simulink model "UNIFIER_ROMdyn_slx"  (R2023b)
settings: Solver=VariableStepAuto  StartTime=0.0  StopTime=0  RelTol=1e-3
InitFcn:
  | UNIFIER_LOAD_ROM
values from neighbouring files (symbols this model uses):
  c = 1.43676    [UNIFIER_LOAD.mat]
  dp_DEP =     [UNIFIER_LOAD.mat]
  dp_HTU =     [UNIFIER_LOAD.mat]
  m = 7057    [UNIFIER_LOAD.mat]
  S = 29.98388    [UNIFIER_LOAD.mat]
  xyz_DEP = [-6.9629998 -10.05 -0.90899998 -6.921 -8.4499998 -0.792 -6.8660002 -6.8499999 -0.82300001 -6.8099999 -5.25 -0.85000002 ... (36 elements, 3x12)]    [UNIFIER_LOAD.mat]
undefined symbols (not defined in the file or in its folder): g, Iyy, ROM, xyz_cg_12
libraries: dspindex x2, simulink x1, aerolibatmos2 x1
settings Model: Creator=Reggie Johanes  LastModifiedBy=Reggie Johanes

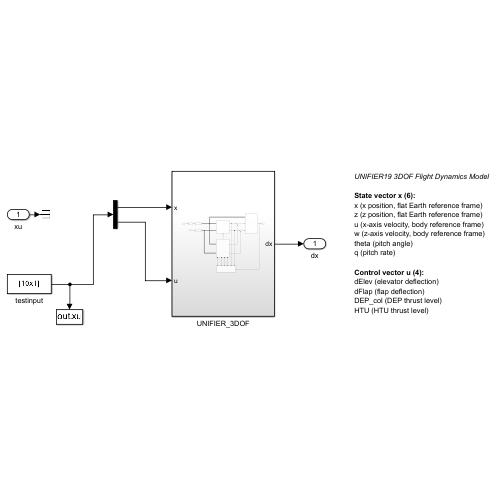
[thumbnail: Simulink's stored preview of the top-level diagram]
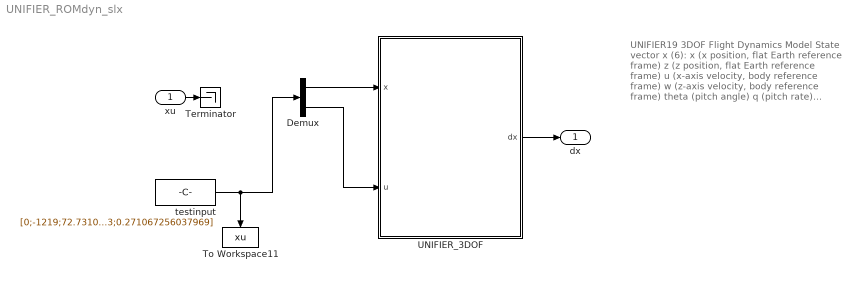
== system UNIFIER_ROMdyn_slx ==
  note: UNIFIER19 3DOF Flight Dynamics Model
      |
      | State vector x (6):
      | x (x position, flat Earth reference frame)
      | z (z position, flat Earth reference frame)
      | u (x-axis velocity, body reference frame)
      | w (z-axis velocity, body reference frame)
      | theta (pitch angle)
      | q (pitch rate)
      |
      | Control vector u (4):
      | dElev (elevator deflection)
      | dFlap (flap deflection)
      | DEP_col (DEP thrust level)
      | HTU (HTU thrust level)
  xu : Inport
  Demux : Demux  Outputs=[6,4]
  Terminator : Terminator
  To Workspace11 : ToWorkspace  VariableName=xu  SampleTime=-1
  UNIFIER_3DOF : Subsystem
  testinput : Constant  Value=[0;-1219;72.731047032614440;1.142307104518741;0.015706052282666;0;-0.015298320692100;0;0.306978739246813;0.271067256037969]
  dx : Outport
  wires:
  UNIFIER_3DOF/1(dx) -> dx/1
  xu/1 -> Terminator/1
  testinput/1 -> To Workspace11/1, Demux/1
  Demux/1 -> UNIFIER_3DOF/1(x)
  Demux/2 -> UNIFIER_3DOF/2(u)

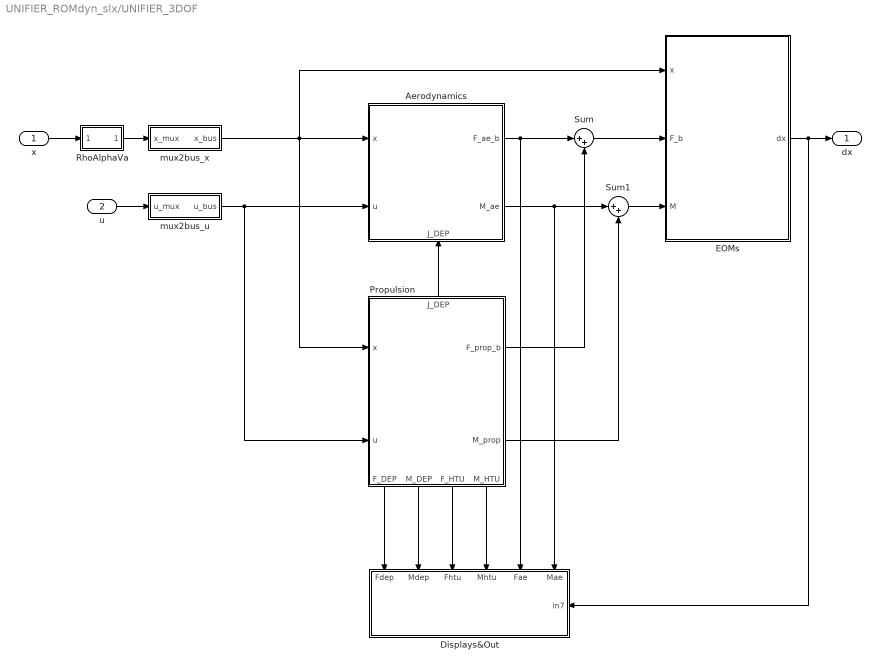
== system UNIFIER_ROMdyn_slx/UNIFIER_3DOF ==
  x : Inport
  u : Inport  Port=2
  Aerodynamics : Subsystem
      settings: PortSchema="{\"entries\":[{\"content\":{\"sides\":[{\"content\":{\"connectorIds\":[\"In1\",\"In2\"]},\"type\":\"ConnectorPlacement.EquallySpacedRectSide\",\"uuid\":\"17ee4459-7bca-4fc7-ac8a-5f8d484d0f96\"},{\"content\":{\"connectorIds\":[\"Out1\",\"Out2\"],\"side\":\"RIGHT\"},\"type\":\"ConnectorPlacement.EquallySpacedRectSide\",\"uuid\":\"9b92559e-06f7-4af4-8484-f34dac8672b4\"},{\"content\":{\"side\":\"TOP\"},\"type\":\"ConnectorPlacement.EquallySpacedRectSide\",\"uuid\":\"a4f2e9fa-eae6-474f-ad2c-489301d84b22\"},{\"content\":{\"connectorIds\":[\"In3\"],\"side\":\"BOTTOM\"},\"type\":\"ConnectorPlacement.EquallySpacedRectSide\",\"uuid\":\"178ea2f1-e4a2-458b-b79e-a56beb6169b5\"}]},\"type\":\"ConnectorPlacement.EquallySpacedConnector\",\"uuid\":\"479c014a-6cba-4ef7-bfe0-51bf14fc9f63\"}],\"packageUris\":[\"http://schema.mathworks.com/mf0/Connector/R2020b\"],\"version\":\"1.0\"}"
  Displays&Out : Subsystem
      settings: PortSchema="{\"entries\":[{\"content\":{\"sides\":[{\"content\":{\"connectorIds\":[\"In1\",\"In2\",\"In3\",\"In4\",\"In5\",\"In6\"]},\"type\":\"ConnectorPlacement.EquallySpacedRectSide\",\"uuid\":\"4905a1e6-f187-42f6-8861-554ce46575dc\"},{\"content\":{\"side\":\"RIGHT\"},\"type\":\"ConnectorPlacement.EquallySpacedRectSide\",\"uuid\":\"de3d9a7f-36bf-4f11-b8b8-ca122b0da870\"},{\"content\":{\"side\":\"TOP\"},\"type\":\"ConnectorPlacement.EquallySpacedRectSide\",\"uuid\":\"fa2b7d06-3d15-496a-b7bf-21f5ef1da56f\"},{\"content\":{\"connectorIds\":[\"In7\"],\"side\":\"BOTTOM\"},\"type\":\"ConnectorPlacement.EquallySpacedRectSide\",\"uuid\":\"8a706778-a274-460f-8ce7-007ff646b71a\"}]},\"type\":\"ConnectorPlacement.EquallySpacedConnector\",\"uuid\":\"cc6e620d-d6cf-4744-801e-d0f26400d64e\"}],\"packageUris\":[\"http://schema.mathworks.com/mf0/Connector/R2020b\"],\"version\":\"1.0\"}"
  EOMs : Subsystem
  Propulsion : Subsystem
      settings: PortSchema="{\"entries\":[{\"content\":{\"sides\":[{\"content\":{\"connectorIds\":[\"In1\",\"In2\"]},\"type\":\"ConnectorPlacement.EquallySpacedRectSide\",\"uuid\":\"07d6f334-da9b-43bc-8919-35c75dc56ebf\"},{\"content\":{\"connectorIds\":[\"Out1\",\"Out2\"],\"side\":\"RIGHT\"},\"type\":\"ConnectorPlacement.EquallySpacedRectSide\",\"uuid\":\"71e67728-3303-46b8-a0cb-58b7e4eaf9eb\"},{\"content\":{\"connectorIds\":[\"Out7\"],\"side\":\"TOP\"},\"type\":\"ConnectorPlacement.EquallySpacedRectSide\",\"uuid\":\"b3b60b63-634a-4790-bc05-b0be525e2f04\"},{\"content\":{\"connectorIds\":[\"Out3\",\"Out4\",\"Out5\",\"Out6\"],\"side\":\"BOTTOM\"},\"type\":\"ConnectorPlacement.EquallySpacedRectSide\",\"uuid\":\"08f8613a-9fde-47a6-8a5d-0759c49fe0b0\"}]},\"type\":\"ConnectorPlacement.EquallySpacedConnector\",\"uuid\":\"5a9d657d-d483-47e8-9c23-43355ba90f0d\"}],\"packageUris\":[\"http://schema.mathworks.com/mf0/Connector/R2020b\"],\"version\":\"1.0\"}"
  RhoAlphaVa : Subsystem
  Sum : Sum  Inputs=|++
  Sum1 : Sum  Inputs=|++
  mux2bus_u : Subsystem
  mux2bus_x : Subsystem
  dx : Outport
  wires:
  u/1 -> mux2bus_u/1(u_mux)
  x/1 -> RhoAlphaVa/1(In1)
  Aerodynamics/1(F_ae_b) -> Displays&Out/5(Fae), Sum/1
  Sum/1 -> EOMs/2(F_b)
  Propulsion/1(F_prop_b) -> Sum/2
  Aerodynamics/2(M_ae) -> Displays&Out/6(Mae), Sum1/1
  Sum1/1 -> EOMs/3(M)
  Propulsion/2(M_prop) -> Sum1/2
  EOMs/1(dx) -> Displays&Out/7(in7), dx/1
  RhoAlphaVa/1(Out1) -> mux2bus_x/1(x_mux)
  mux2bus_x/1(x_bus) -> EOMs/1(x), Aerodynamics/1(x), Propulsion/1(x)
  mux2bus_u/1(u_bus) -> Aerodynamics/2(u), Propulsion/2(u)
  Propulsion/7(J_DEP) -> Aerodynamics/3(J_DEP)
  Propulsion/3(F_DEP) -> Displays&Out/1(Fdep)
  Propulsion/4(M_DEP) -> Displays&Out/2(Mdep)
  Propulsion/5(F_HTU) -> Displays&Out/3(Fhtu)
  Propulsion/6(M_HTU) -> Displays&Out/4(Mhtu)

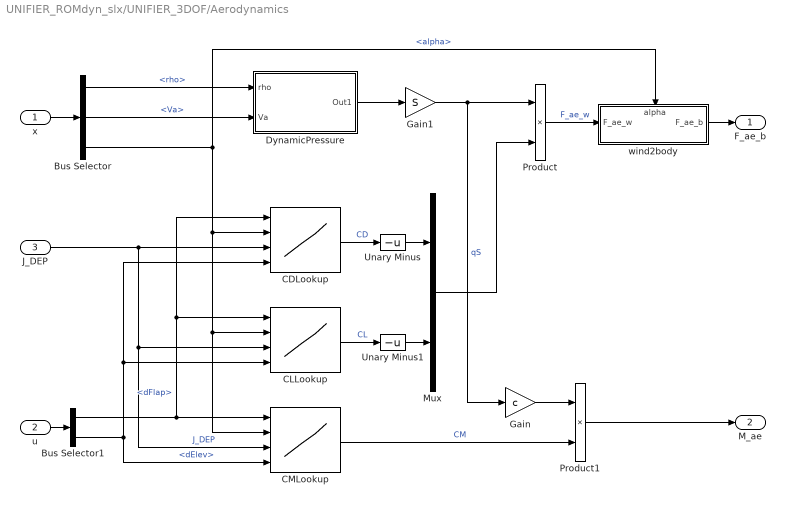
== system UNIFIER_ROMdyn_slx/UNIFIER_3DOF/Aerodynamics ==
  x : Inport
  u : Inport  Port=2
  J_DEP : Inport  Port=3
  Bus Selector : BusSelector  OutputSignals=rho,Va,alpha
  Bus Selector1 : BusSelector  OutputSignals=dFlap,dElev
  CDLookup : Lookup_n-D  NumberOfTableDimensions=4  BreakpointsForDimension1=ROM.dFlap  BreakpointsForDimension2=ROM.alpha  BreakpointsForDimension3=ROM.J  BreakpointsForDimension4=ROM.dElev  Table=ROM.CD  ExtrapMethod=Clip  UseLastTableValue=on  InternalRulePriority=Speed  RndMeth=Simplest
      settings: InputPortMap=u0,u1,u2,u3
  CLLookup : Lookup_n-D  NumberOfTableDimensions=4  BreakpointsForDimension1=ROM.dFlap  BreakpointsForDimension2=ROM.alpha  BreakpointsForDimension3=ROM.J  BreakpointsForDimension4=ROM.dElev  Table=ROM.CL  ExtrapMethod=Clip  UseLastTableValue=on  InternalRulePriority=Speed  RndMeth=Simplest
      settings: InputPortMap=u0,u1,u2,u3
  CMLookup : Lookup_n-D  NumberOfTableDimensions=4  BreakpointsForDimension1=ROM.dFlap  BreakpointsForDimension2=ROM.alpha  BreakpointsForDimension3=ROM.J  BreakpointsForDimension4=ROM.dElev  Table=ROM.CM  ExtrapMethod=Clip  UseLastTableValue=on  InternalRulePriority=Speed  RndMeth=Simplest
      settings: InputPortMap=u0,u1,u2,u3
  DynamicPressure : Subsystem
  Gain : Gain  Gain=c
  Gain1 : Gain  Gain=S
  Mux : Mux  Inputs=2
  Product : Product
  Product1 : Product
  Unary Minus : UnaryMinus
  Unary Minus1 : UnaryMinus
  wind2body : Subsystem
      settings: PortSchema="{\"entries\":[{\"content\":{\"sides\":[{\"content\":{\"connectorIds\":[\"In1\"]},\"type\":\"ConnectorPlacement.EquallySpacedRectSide\",\"uuid\":\"290c73ed-3dea-48ea-8152-da6c73d4cb7e\"},{\"content\":{\"connectorIds\":[\"Out1\"],\"side\":\"RIGHT\"},\"type\":\"ConnectorPlacement.EquallySpacedRectSide\",\"uuid\":\"998f7612-46b2-4329-a1d2-339c41b842ac\"},{\"content\":{\"connectorIds\":[\"In2\"],\"side\":\"TOP\"},\"type\":\"ConnectorPlacement.EquallySpacedRectSide\",\"uuid\":\"f5aa2474-eb99-4d6b-9b61-1c1ef88f9e9d\"}]},\"type\":\"ConnectorPlacement.EquallySpacedConnector\",\"uuid\":\"e9cadda8-b54c-4a15-b91d-81264397230a\"}],\"packageUris\":[\"http://schema.mathworks.com/mf0/Connector/R2020b\"],\"version\":\"1.0\"}"
  F_ae_b : Outport
  M_ae : Outport  Port=2
  wires:
  x/1 -> Bus Selector/1
  DynamicPressure/1(Out1) -> Gain1/1
  u/1 -> Bus Selector1/1
  Bus Selector1/1 -> CMLookup/1, CDLookup/1, CLLookup/1  "<dFlap>"
  Bus Selector/2 -> DynamicPressure/2(Va)  "<Va>"
  Bus Selector/1 -> DynamicPressure/1(rho)  "<rho>"
  Bus Selector/3 -> wind2body/2(alpha), CMLookup/2, CLLookup/2, CDLookup/2  "<alpha>"
  Gain1/1 -> Gain/1, Product/1  "qS"
  Bus Selector1/2 -> CMLookup/4, CDLookup/4, CLLookup/4  "<dElev>"
  J_DEP/1 -> CMLookup/3, CLLookup/3, CDLookup/3  "J_DEP"
  CDLookup/1 -> Unary Minus/1  "CD"
  Product/1 -> wind2body/1(F_ae_w)  "F_ae_w"
  CLLookup/1 -> Unary Minus1/1  "CL"
  Unary Minus/1 -> Mux/1
  Unary Minus1/1 -> Mux/2
  Mux/1 -> Product/2
  wind2body/1(F_ae_b) -> F_ae_b/1
  CMLookup/1 -> Product1/2  "CM"
  Gain/1 -> Product1/1
  Product1/1 -> M_ae/1

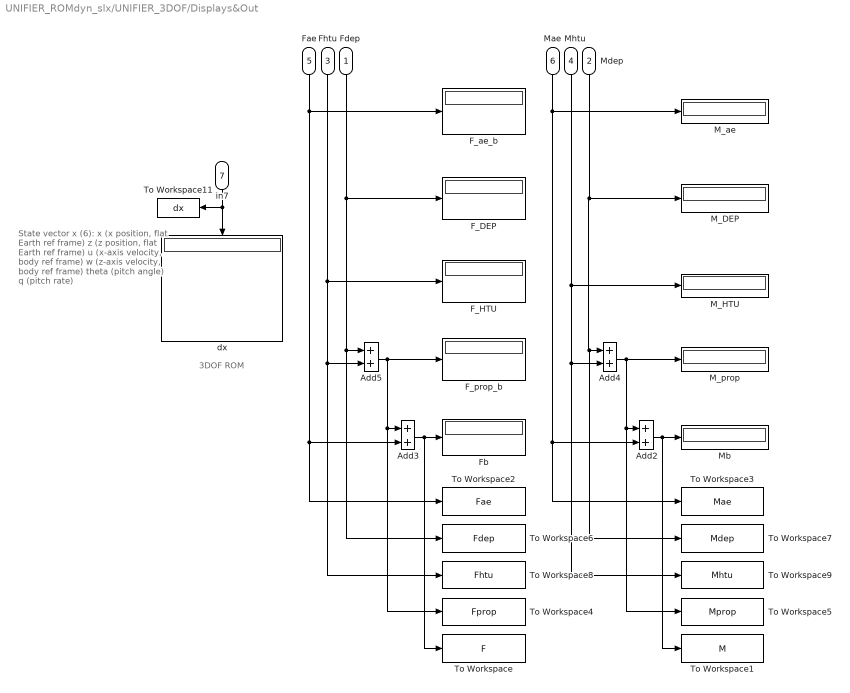
== system UNIFIER_ROMdyn_slx/UNIFIER_3DOF/Displays&Out ==
  note: 3DOF ROM
  note: State vector x (6):
      | x (x position, flat Earth ref frame)
      | z (z position, flat Earth ref frame)
      | u (x-axis velocity, body ref frame)
      | w (z-axis velocity, body ref frame)
      | theta (pitch angle)
      | q (pitch rate)
  Fdep : Inport
  Mdep : Inport  Port=2
  Fhtu : Inport  Port=3
  Mhtu : Inport  Port=4
  Fae : Inport  Port=5
  Mae : Inport  Port=6
  in7 : Inport  Port=7
  Add{2..5} (4 alike) : Sum
  F_DEP : Display
  F_HTU : Display
  F_ae_b : Display
  F_prop_b : Display
  Fb : Display
  M_DEP : Display
  M_HTU : Display
  M_ae : Display
  M_prop : Display
  Mb : Display
  To Workspace : ToWorkspace  VariableName=F  SampleTime=-1
  To Workspace1 : ToWorkspace  VariableName=M  SampleTime=-1
  To Workspace11 : ToWorkspace  VariableName=dx  SampleTime=-1
  To Workspace2 : ToWorkspace  VariableName=Fae  SampleTime=-1
  To Workspace3 : ToWorkspace  VariableName=Mae  SampleTime=-1
  To Workspace4 : ToWorkspace  VariableName=Fprop  SampleTime=-1
  To Workspace5 : ToWorkspace  VariableName=Mprop  SampleTime=-1
  To Workspace6 : ToWorkspace  VariableName=Fdep  SampleTime=-1
  To Workspace7 : ToWorkspace  VariableName=Mdep  SampleTime=-1
  To Workspace8 : ToWorkspace  VariableName=Fhtu  SampleTime=-1
  To Workspace9 : ToWorkspace  VariableName=Mhtu  SampleTime=-1
  dx : Display
  wires:
  Fae/1 -> F_ae_b/1, Add3/2, To Workspace2/1
  Mae/1 -> Add2/2, To Workspace3/1, M_ae/1
  Fhtu/1 -> F_HTU/1, Add5/2, To Workspace8/1
  Mdep/1 -> M_DEP/1, To Workspace7/1, Add4/1
  Mhtu/1 -> M_HTU/1, Add4/2, To Workspace9/1
  Fdep/1 -> F_DEP/1, Add5/1, To Workspace6/1
  Add3/1 -> To Workspace/1, Fb/1
  Add2/1 -> To Workspace1/1, Mb/1
  Add4/1 -> To Workspace5/1, Add2/1, M_prop/1
  Add5/1 -> F_prop_b/1, To Workspace4/1, Add3/1
  in7/1 -> dx/1, To Workspace11/1

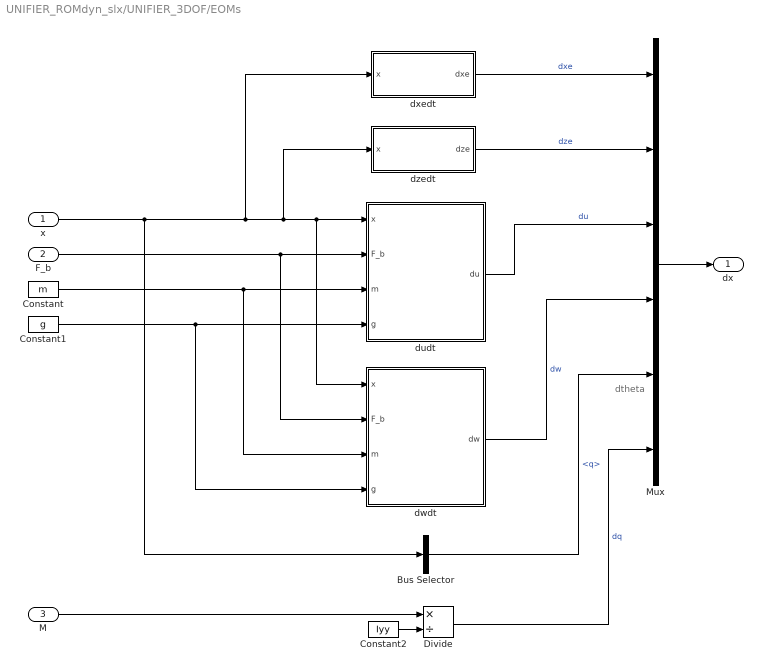
== system UNIFIER_ROMdyn_slx/UNIFIER_3DOF/EOMs ==
  note: dtheta
  x : Inport
  F_b : Inport  Port=2
  M : Inport  Port=3
  Bus Selector : BusSelector  OutputSignals=q
  Constant : Constant  Value=m
  Constant1 : Constant  Value=g
  Constant2 : Constant  Value=Iyy
  Divide : Product  Inputs=*/
  Mux : Mux  Inputs=6
  dudt : Subsystem
  dwdt : Subsystem
  dxedt : Subsystem
  dzedt : Subsystem
  dx : Outport
  wires:
  M/1 -> Divide/1
  Constant2/1 -> Divide/2
  Mux/1 -> dx/1
  Divide/1 -> Mux/6  "dq"
  x/1 -> Bus Selector/1, dxedt/1(x), dzedt/1(x), dwdt/1(x), dudt/1(x)
  F_b/1 -> dwdt/2(F_b), dudt/2(F_b)
  Constant/1 -> dwdt/3(m), dudt/3(m)
  Constant1/1 -> dwdt/4(g), dudt/4(g)
  dudt/1(du) -> Mux/3  "du"
  dxedt/1(dxe) -> Mux/1  "dxe"
  dzedt/1(dze) -> Mux/2  "dze"
  dwdt/1(dw) -> Mux/4  "dw"
  Bus Selector/1 -> Mux/5  "<q>"

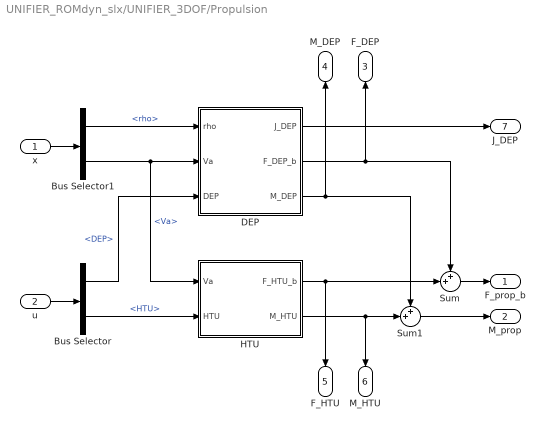
== system UNIFIER_ROMdyn_slx/UNIFIER_3DOF/Propulsion ==
  x : Inport
  u : Inport  Port=2
  Bus Selector : BusSelector  OutputSignals=DEP,HTU
  Bus Selector1 : BusSelector  OutputSignals=rho,Va
  DEP : Subsystem
  HTU : Subsystem
  Sum : Sum  Inputs=++|
  Sum1 : Sum  Inputs=++|
  F_prop_b : Outport
  M_prop : Outport  Port=2
  F_DEP : Outport  Port=3
  M_DEP : Outport  Port=4
  F_HTU : Outport  Port=5
  M_HTU : Outport  Port=6
  J_DEP : Outport  Port=7
  wires:
  u/1 -> Bus Selector/1
  x/1 -> Bus Selector1/1
  Bus Selector1/2 -> HTU/1(Va), DEP/2(Va)  "<Va>"
  Bus Selector/1 -> DEP/3(DEP)  "<DEP>"
  Bus Selector/2 -> HTU/2(HTU)  "<HTU>"
  DEP/1(J_DEP) -> J_DEP/1
  HTU/2(M_HTU) -> Sum1/2, M_HTU/1
  HTU/1(F_HTU_b) -> Sum/2, F_HTU/1
  DEP/2(F_DEP_b) -> Sum/1, F_DEP/1
  DEP/3(M_DEP) -> Sum1/1, M_DEP/1
  Sum/1 -> F_prop_b/1
  Sum1/1 -> M_prop/1
  Bus Selector1/1 -> DEP/1(rho)  "<rho>"

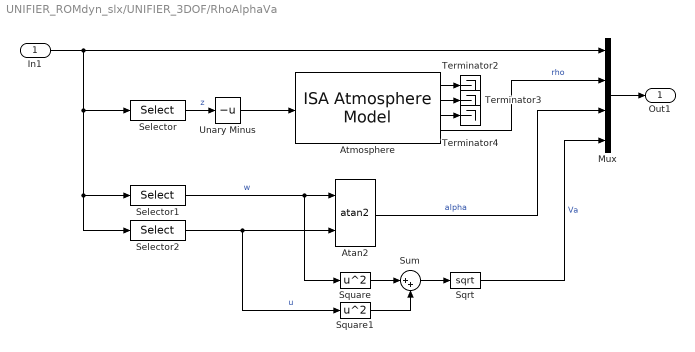
== system UNIFIER_ROMdyn_slx/UNIFIER_3DOF/RhoAlphaVa ==
  In1 : Inport
  Atan2 : Trigonometry  Operator=atan2
  Atmosphere : aerolibatmos2/ISA Atmosphere Model  useExtended=off  action=Warning  custom=off  viscosityOut=off  g=9.80665  gamma=1.4  R=287.0531  L=0.0065  h_trop=11000  h_strat=20000  rho0=1.225  P0=101325  T0=288.15  h0=0
  Mux : Mux
  Selector : Selector  InputPortWidth=6  IndexOptions=Index vector (dialog)  Indices=2  OutputSizes=1
  Selector1 : Selector  InputPortWidth=6  IndexOptions=Index vector (dialog)  Indices=4  OutputSizes=1
  Selector2 : Selector  InputPortWidth=6  IndexOptions=Index vector (dialog)  Indices=3  OutputSizes=1
  Sqrt : Sqrt
  Square : Math  Operator=square
  Square1 : Math  Operator=square
  Sum : Sum  Inputs=|++
  Terminator2 : Terminator
  Terminator3 : Terminator
  Terminator4 : Terminator
  Unary Minus : UnaryMinus
  Out1 : Outport
  wires:
  In1/1 -> Selector2/1, Selector1/1, Selector/1, Mux/1
  Selector/1 -> Unary Minus/1  "z"
  Unary Minus/1 -> Atmosphere/1
  Atmosphere/3 -> Terminator4/1
  Atmosphere/4 -> Mux/2  "rho"
  Atmosphere/2 -> Terminator3/1
  Atmosphere/1 -> Terminator2/1
  Mux/1 -> Out1/1
  Selector2/1 -> Square1/1, Atan2/2  "u"
  Atan2/1 -> Mux/3  "alpha"
  Sum/1 -> Sqrt/1
  Square1/1 -> Sum/2
  Selector1/1 -> Square/1, Atan2/1  "w"
  Square/1 -> Sum/1
  Sqrt/1 -> Mux/4  "Va"

== system UNIFIER_ROMdyn_slx/UNIFIER_3DOF/mux2bus_u ==
  u_mux : Inport
  Bus Creator : BusCreator  Inputs=4
  Demux : Demux
  u_bus : Outport
  wires:
  u_mux/1 -> Demux/1
  Demux/2 -> Bus Creator/2  "dFlap"
  Demux/3 -> Bus Creator/3  "DEP"
  Demux/1 -> Bus Creator/1  "dElev"
  Bus Creator/1 -> u_bus/1
  Demux/4 -> Bus Creator/4  "HTU"

== system UNIFIER_ROMdyn_slx/UNIFIER_3DOF/mux2bus_x ==
  x_mux : Inport
  Bus Creator : BusCreator  Inputs=9
  Demux : Demux  Outputs=9
  x_bus : Outport
  wires:
  x_mux/1 -> Demux/1
  Bus Creator/1 -> x_bus/1
  Demux/1 -> Bus Creator/1  "xe"
  Demux/2 -> Bus Creator/2  "ze"
  Demux/3 -> Bus Creator/3  "u"
  Demux/4 -> Bus Creator/4  "w"
  Demux/5 -> Bus Creator/5  "theta"
  Demux/6 -> Bus Creator/6  "q"
  Demux/7 -> Bus Creator/7  "rho"
  Demux/8 -> Bus Creator/8  "alpha"
  Demux/9 -> Bus Creator/9  "Va"

== system UNIFIER_ROMdyn_slx/UNIFIER_3DOF/Aerodynamics/DynamicPressure ==
  rho : Inport
  Va : Inport  Port=2
  Gain : Gain  Gain=0.5
  Product : Product
  Square : Math  Operator=square
  Out1 : Outport
  wires:
  Va/1 -> Square/1
  rho/1 -> Gain/1
  Square/1 -> Product/1
  Gain/1 -> Product/2
  Product/1 -> Out1/1

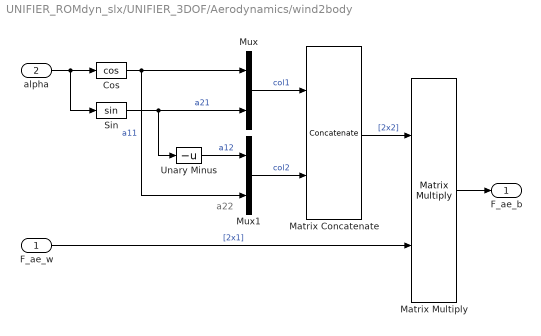
== system UNIFIER_ROMdyn_slx/UNIFIER_3DOF/Aerodynamics/wind2body ==
  note: a22
  F_ae_w : Inport
  alpha : Inport  Port=2
  Cos : Trigonometry  Operator=cos
  Matrix Concatenate : Concatenate  Mode=Multidimensional array  ConcatenateDimension=2
  Matrix Multiply : Product  Multiplication=Matrix(*)
  Mux : Mux  Inputs=2
  Mux1 : Mux  Inputs=2
  Sin : Trigonometry
  Unary Minus : UnaryMinus
  F_ae_b : Outport
  wires:
  alpha/1 -> Sin/1, Cos/1
  Matrix Concatenate/1 -> Matrix Multiply/1  "[2x2]"
  F_ae_w/1 -> Matrix Multiply/2  "[2x1]"
  Matrix Multiply/1 -> F_ae_b/1
  Mux/1 -> Matrix Concatenate/1  "col1"
  Mux1/1 -> Matrix Concatenate/2  "col2"
  Unary Minus/1 -> Mux1/1  "a12"
  Cos/1 -> Mux/1, Mux1/2  "a11"
  Sin/1 -> Mux/2, Unary Minus/1  "a21"

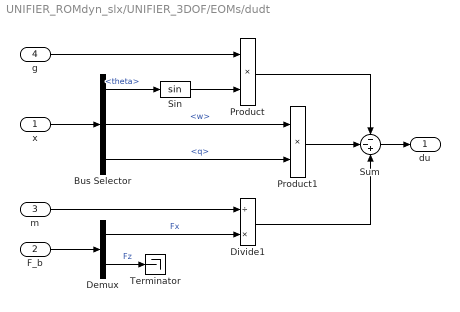
== system UNIFIER_ROMdyn_slx/UNIFIER_3DOF/EOMs/dudt ==
  x : Inport
  F_b : Inport  Port=2
  m : Inport  Port=3
  g : Inport  Port=4
  Bus Selector : BusSelector  OutputSignals=theta,w,q
  Demux : Demux  Outputs=2
  Divide1 : Product  Inputs=/*
  Product : Product
  Product1 : Product
  Sin : Trigonometry
  Sum : Sum  Inputs=--+
  Terminator : Terminator
  du : Outport
  wires:
  Product/1 -> Sum/1
  Sin/1 -> Product/2
  Bus Selector/2 -> Product1/1  "<w>"
  Bus Selector/1 -> Sin/1  "<theta>"
  Bus Selector/3 -> Product1/2  "<q>"
  Product1/1 -> Sum/2
  Demux/2 -> Terminator/1  "Fz"
  x/1 -> Bus Selector/1
  F_b/1 -> Demux/1
  g/1 -> Product/1
  m/1 -> Divide1/1
  Sum/1 -> du/1
  Demux/1 -> Divide1/2  "Fx"
  Divide1/1 -> Sum/3

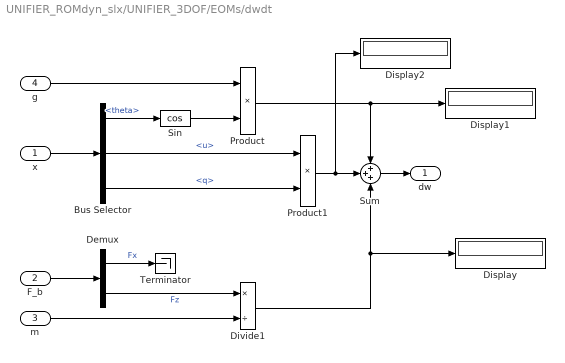
== system UNIFIER_ROMdyn_slx/UNIFIER_3DOF/EOMs/dwdt ==
  x : Inport
  F_b : Inport  Port=2
  m : Inport  Port=3
  g : Inport  Port=4
  Bus Selector : BusSelector  OutputSignals=theta,u,q
  Demux : Demux  Outputs=2
  Display : Display
  Display1 : Display
  Display2 : Display
  Divide1 : Product  Inputs=*/
  Product : Product
  Product1 : Product
  Sin : Trigonometry  Operator=cos
  Sum : Sum  Inputs=+++
  Terminator : Terminator
  dw : Outport
  wires:
  Product/1 -> Sum/1, Display1/1
  Sin/1 -> Product/2
  Bus Selector/2 -> Product1/1  "<u>"
  Bus Selector/1 -> Sin/1  "<theta>"
  Bus Selector/3 -> Product1/2  "<q>"
  Product1/1 -> Display2/1, Sum/2
  Demux/2 -> Divide1/1  "Fz"
  x/1 -> Bus Selector/1
  F_b/1 -> Demux/1
  g/1 -> Product/1
  m/1 -> Divide1/2
  Sum/1 -> dw/1
  Demux/1 -> Terminator/1  "Fx"
  Divide1/1 -> Display/1, Sum/3

== system UNIFIER_ROMdyn_slx/UNIFIER_3DOF/EOMs/dxedt ==
  x : Inport
  Bus Selector : BusSelector  OutputSignals=u,w,theta
  Cos : Trigonometry  Operator=cos
  Cos1 : Trigonometry
  Product : Product
  Product1 : Product
  Sum : Sum  Inputs=|++
  dxe : Outport
  wires:
  x/1 -> Bus Selector/1
  Bus Selector/1 -> Product1/1  "<u>"
  Bus Selector/2 -> Product/1  "<w>"
  Bus Selector/3 -> Cos/1, Cos1/1  "<theta>"
  Cos1/1 -> Product/2
  Cos/1 -> Product1/2
  Product/1 -> Sum/2
  Product1/1 -> Sum/1
  Sum/1 -> dxe/1

== system UNIFIER_ROMdyn_slx/UNIFIER_3DOF/EOMs/dzedt ==
  x : Inport
  Bus Selector : BusSelector  OutputSignals=u,w,theta
  Cos : Trigonometry
  Cos1 : Trigonometry  Operator=cos
  Product : Product
  Product1 : Product
  Sum : Sum  Inputs=|-+
  dze : Outport
  wires:
  x/1 -> Bus Selector/1
  Bus Selector/1 -> Product1/1  "<u>"
  Bus Selector/2 -> Product/1  "<w>"
  Bus Selector/3 -> Cos/1, Cos1/1  "<theta>"
  Cos1/1 -> Product/2
  Cos/1 -> Product1/2
  Product/1 -> Sum/2
  Product1/1 -> Sum/1
  Sum/1 -> dze/1

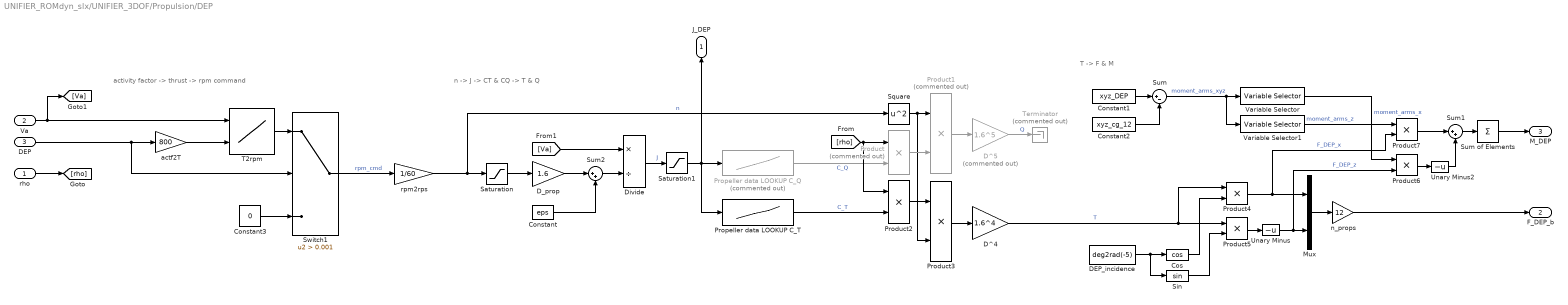
== system UNIFIER_ROMdyn_slx/UNIFIER_3DOF/Propulsion/DEP ==
  note: T -> F & M
  note: n -> J -> CT & CQ -> T & Q
  note: activity factor -> thrust -> rpm command
  rho : Inport
  Va : Inport  Port=2
  DEP : Inport  Port=3
  Constant : Constant  Value=eps
  Constant1 : Constant  Value=xyz_DEP
  Constant2 : Constant  Value=xyz_cg_12
  Constant3 : Constant  Value=0
  Cos : Trigonometry  Operator=cos
  DEP_incidence : Constant  Value=deg2rad(-5)
  D^4 : Gain  Gain=1.6^4
  D^5 : Gain  Commented=on  Gain=1.6^5
  D_prop : Gain  Gain=1.6
  Divide : Product  Inputs=*/
  Mux : Mux  Inputs=2
  Product : Product  Commented=on
  Product1 : Product  Commented=on
  Product{2..7} (6 alike) : Product
  Propeller data LOOKUP C_Q : Lookup_n-D  Commented=on  NumberOfTableDimensions=1  BreakpointsForDimension1=dp_DEP.J  IndexSearchMethod=Linear search  BeginIndexSearchUsingPreviousIndexResult=on  Table=dp_DEP.C_Q  ExtrapMethod=Clip  UseLastTableValue=on  InternalRulePriority=Speed  RndMeth=Simplest
  Propeller data LOOKUP C_T : Lookup_n-D  NumberOfTableDimensions=1  BreakpointsForDimension1=dp_DEP.J  IndexSearchMethod=Linear search  BeginIndexSearchUsingPreviousIndexResult=on  Table=dp_DEP.C_T  ExtrapMethod=Clip  UseLastTableValue=on  InternalRulePriority=Speed  RndMeth=Simplest
  Saturation : Saturate  UpperLimit=inf  LowerLimit=0
  Saturation1 : Saturate  UpperLimit=2.5  LowerLimit=0.3
  Sin : Trigonometry
  Square : Math  Operator=square
  Sum : Sum  Inputs=|+-
  Sum of Elements : Sum  Inputs=+
  Sum1 : Sum  Inputs=|++
  Sum2 : Sum  Inputs=|++
  Switch1 : Switch  Criteria=u2 > Threshold  Threshold=0.001  SaturateOnIntegerOverflow=off  InputSameDT=off
  T2rpm : Lookup_n-D  BreakpointsForDimension1=dp_DEP.rpm_lookup.V_vec  BreakpointsForDimension2=dp_DEP.rpm_lookup.T_vec  IndexSearchMethod=Linear search  BeginIndexSearchUsingPreviousIndexResult=on  Table=dp_DEP.rpm_lookup.rpm_gird  ExtrapMethod=Clip  InternalRulePriority=Speed  RndMeth=Simplest
      settings: InputPortMap=u0,u1
  Terminator : Terminator  Commented=on
  Unary Minus : UnaryMinus
  Unary Minus2 : UnaryMinus
  Variable Selector : dspindex/Variable Selector  NumInputs=1  rowsOrCols=Rows  IdxMode=Fixed  Elements=[1]  ZerOneIdxMode=One-based  errmode=Clip Index  FillMode=off  FillValues=0
  Variable Selector1 : dspindex/Variable Selector  NumInputs=1  rowsOrCols=Rows  IdxMode=Fixed  Elements=[3]  ZerOneIdxMode=One-based  errmode=Clip Index  FillMode=off  FillValues=0
  actf2T : Gain  Gain=800
  n_props : Gain  Gain=12
  rpm2rps : Gain  Gain=1/60
  J_DEP : Outport
  F_DEP_b : Outport  Port=2
  M_DEP : Outport  Port=3
  wires:
  Constant3/1 -> Switch1/3
  DEP/1 -> actf2T/1, Switch1/2
  actf2T/1 -> T2rpm/2
  T2rpm/1 -> Switch1/1
  Va/1 -> [Va], T2rpm/1
  Switch1/1 -> rpm2rps/1  "rpm_cmd"
  rho/1 -> [rho]
  [Va] -> Divide/1
  Constant/1 -> Sum2/2
  Divide/1 -> Saturation1/1  "J"
  D_prop/1 -> Sum2/1
  Sum2/1 -> Divide/2
  Saturation/1 -> D_prop/1
  rpm2rps/1 -> Square/1, Saturation/1  "n"
  Saturation1/1 -> Propeller data LOOKUP C_Q/1, Propeller data LOOKUP C_T/1, J_DEP/1
  Propeller data LOOKUP C_Q/1 -> Product/2  "C_Q"
  Propeller data LOOKUP C_T/1 -> Product2/2  "C_T"
  [rho] -> Product2/1, Product/1
  Square/1 -> Product1/1, Product3/2
  Product/1 -> Product1/2
  D^5/1 -> Terminator/1  "Q"
  D^4/1 -> Product4/1, Product5/1  "T"
  Product1/1 -> D^5/1
  Product3/1 -> D^4/1
  Product2/1 -> Product3/1
  DEP_incidence/1 -> Sin/1, Cos/1
  Cos/1 -> Product4/2
  Sin/1 -> Product5/2
  Product5/1 -> Unary Minus/1
  n_props/1 -> F_DEP_b/1
  Constant1/1 -> Sum/1
  Constant2/1 -> Sum/2
  Sum/1 -> Variable Selector/1, Variable Selector1/1  "moment_arms_xyz"
  Variable Selector/1 -> Product6/1  "moment_arms_x"
  Variable Selector1/1 -> Product7/1  "moment_arms_z"
  Mux/1 -> n_props/1
  Unary Minus/1 -> Product6/2, Mux/2  "F_DEP_z"
  Product6/1 -> Unary Minus2/1
  Product7/1 -> Sum1/1
  Sum1/1 -> Sum of Elements/1
  Sum of Elements/1 -> M_DEP/1
  Unary Minus2/1 -> Sum1/2
  Product4/1 -> Product7/2, Mux/1  "F_DEP_x"

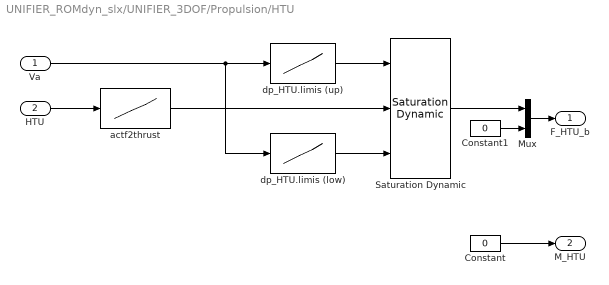
== system UNIFIER_ROMdyn_slx/UNIFIER_3DOF/Propulsion/HTU ==
  Va : Inport
  HTU : Inport  Port=2
  Constant : Constant  Value=0
  Constant1 : Constant  Value=0
  Mux : Mux  Inputs=2
  Saturation Dynamic : simulink/Discontinuities/Saturation Dynamic  OutMin=[]  OutMax=[]  OutDataTypeStr=Inherit: Same as second input  OutDataType=fixdt(1, 16)  OutScaling=2^-10  DoSatur=off
  actf2thrust : Lookup_n-D  NumberOfTableDimensions=1  BreakpointsForDimension1=[-0.5,1.5]  IndexSearchMethod=Linear search  BeginIndexSearchUsingPreviousIndexResult=on  Table=[-5000, 15000]  ExtrapMethod=Clip  InternalRulePriority=Speed  RndMeth=Simplest
  dp_HTU.limis (low) : Lookup_n-D  NumberOfTableDimensions=1  BreakpointsForDimension1=dp_HTU.limits.V_low_lim  IndexSearchMethod=Linear search  BeginIndexSearchUsingPreviousIndexResult=on  Table=dp_HTU.limits.T_low_lim  InternalRulePriority=Speed  RndMeth=Simplest
  dp_HTU.limis (up) : Lookup_n-D  NumberOfTableDimensions=1  BreakpointsForDimension1=dp_HTU.limits.V_up_lim  IndexSearchMethod=Linear search  BeginIndexSearchUsingPreviousIndexResult=on  Table=dp_HTU.limits.T_up_lim  InternalRulePriority=Speed  RndMeth=Simplest
  F_HTU_b : Outport
  M_HTU : Outport  Port=2
  wires:
  Constant/1 -> M_HTU/1
  HTU/1 -> actf2thrust/1
  dp_HTU.limis (low)/1 -> Saturation Dynamic/3
  actf2thrust/1 -> Saturation Dynamic/2
  Saturation Dynamic/1 -> Mux/1
  dp_HTU.limis (up)/1 -> Saturation Dynamic/1
  Va/1 -> dp_HTU.limis (low)/1, dp_HTU.limis (up)/1
  Mux/1 -> F_HTU_b/1
  Constant1/1 -> Mux/2
